simulink model "scheme2"  (R2021a)
settings: Solver=FixedStepAuto  StartTime=0.0  StopTime=20  FixedStep=Tp  RelTol=1e-3
values from neighbouring files (symbols this model uses):
  k = 6    [exercise4.m]
  kp = 1.6    [exercise4.m]
  T_1 = 5.9    [exercise4.m]
  T_2 = 0.8    [exercise4.m]
  Td = 0.08    [exercise4.m]
  Ti = 6    [exercise4.m]
settings Model: Creator=MPatr  LastModifiedBy=Paweł
settings SolverCC: AlgebraicLoopSolver=TrustRegion
settings DebuggingCC: SFMachineParentedDataDiag=warning
settings SFSimCC: CustomCodeUndefinedFunction=UseInterfaceOnly

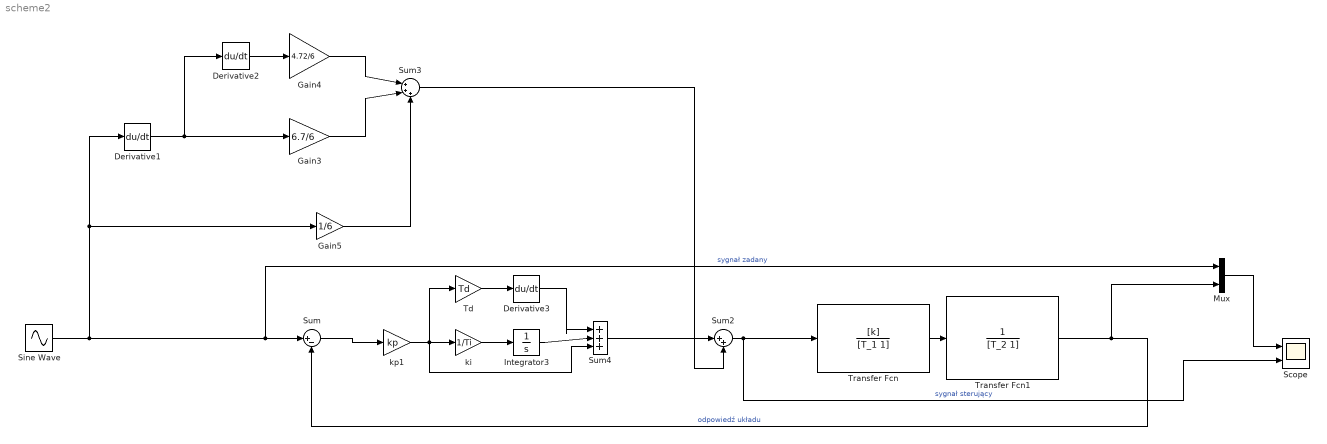
== system scheme2 ==
  Derivative1 : Derivative
  Derivative2 : Derivative
  Derivative3 : Derivative
  Gain3 : Gain  Gain=6.7/6
  Gain4 : Gain  Gain=4.72/6
  Gain5 : Gain  Gain=1/6
  Integrator3 : Integrator
  Mux : Mux  Inputs=2
  Scope : Scope  NumInputPorts=2
  Sine Wave : Sin  Frequency=2  SampleTime=0
  Sum : Sum  Inputs=|+-
  Sum2 : Sum  Inputs=|++
  Sum3 : Sum  Inputs=|+++
  Sum4 : Sum  Inputs=|+++  SaturateOnIntegerOverflow=on
  Td : Gain  Gain=Td  SaturateOnIntegerOverflow=on  OutDataTypeStr=Inherit: Same as input  ParamDataTypeStr=Inherit: Same as input
  Transfer Fcn : TransferFcn  Numerator=[k]  Denominator=[T_1 1]
  Transfer Fcn1 : TransferFcn  Denominator=[T_2 1]
  ki : Gain  Gain=1/Ti  SaturateOnIntegerOverflow=on  OutDataTypeStr=Inherit: Same as input  ParamDataTypeStr=Inherit: Same as input
  kp1 : Gain  Gain=kp  SaturateOnIntegerOverflow=on  OutDataTypeStr=Inherit: Same as input  ParamDataTypeStr=Inherit: Same as input
  wires:
  Transfer Fcn1/1 -> Mux/2, Sum/2  "odpowiedź układu"
  Mux/1 -> Scope/1
  Transfer Fcn/1 -> Transfer Fcn1/1
  Derivative2/1 -> Gain4/1
  Sine Wave/1 -> Gain5/1, Derivative1/1, Mux/1, Sum/1  "sygnał zadany"
  Sum2/1 -> Transfer Fcn/1, Scope/2  "sygnał sterujący"
  Sum3/1 -> Sum2/2
  Gain5/1 -> Sum3/3
  Derivative1/1 -> Derivative2/1, Gain3/1
  Gain4/1 -> Sum3/1
  Gain3/1 -> Sum3/2
  ki/1 -> Integrator3/1
  Derivative3/1 -> Sum4/1
  kp1/1 -> Td/1, Sum4/3, ki/1
  Td/1 -> Derivative3/1
  Integrator3/1 -> Sum4/2
  Sum4/1 -> Sum2/1
  Sum/1 -> kp1/1
